simulink library "Control_Lib"  (R2018a)
settings: Solver=VariableStepAuto  StartTime=0.0  StopTime=10.0  RelTol=1e-3
undefined symbols (not defined in the file or in its folder): fb, Theta0, Tr_PLL
libraries: $bdroot x2, simulink x2
settings Model: Creator=Frederic_Colas  LastModifiedBy=fcolas

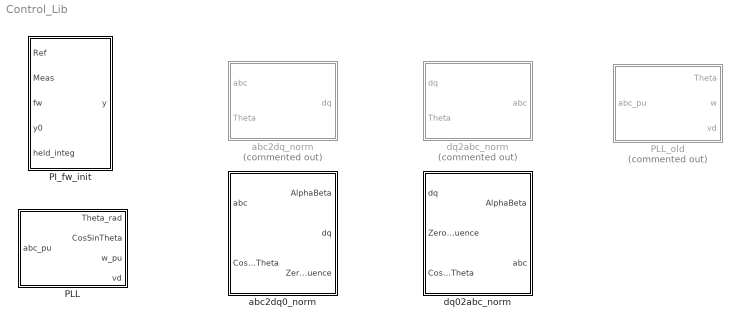
== system Control_Lib ==
  PI_fw_init : Subsystem  TreatAsAtomicUnit=on  mask{Kp=1, Ki=1}
  PLL : Subsystem  TreatAsAtomicUnit=on  mask{fb=fb, Tr_PLL=Tr_PLL, Theta0=Theta0}
      mask prompts: fb "fb (Hz)"; Tr_PLL "PLL time response (ms)"; Theta0 "Theta0 (°)"
      mask init:
      | wb = 2*pi*fb;
      | wn_PLL=5/(Tr_PLL/1000);
      | zeta_PLL = 1;
      | Kp_PLL = 2*zeta_PLL*wn_PLL/wb;
      | Ki_PLL = wn_PLL^2/wb;
  PLL_old : Subsystem  Commented=on  TreatAsAtomicUnit=on  mask{fb=50, Tr_PLL=10, zeta_PLL=1, Theta0=0}
      mask prompts: fb "fb (Hz)"; Tr_PLL "PLL time response (ms)"; zeta_PLL "Damping factor"; Theta0 "Theta0 (°)"
      mask init:
      | wb = 2*pi*fb;
      | wn_PLL=5/(Tr_PLL/1000);
      | zeta_PLL = 1;
      | Kp_PLL = 2*zeta_PLL*wn_PLL/wb;
      | Ki_PLL = wn_PLL^2/wb;
  abc2dq0_norm : Subsystem  TreatAsAtomicUnit=on  mask{referenceAxisMode=Reference axis at 90 degrees behind phase_a, baseUpdateGain=1/sqrt(3)}
      mask prompts: referenceAxisMode "Chosse reference axis of the angular position"; baseUpdateGain "Gain to update base from abc to dq0 frames"
      mask init:
      | Concordia33 = sqrt(2/3)*[[cos(0) cos(-2*pi/3) cos(-4*pi/3)];
      |                  [-sin(0) -sin(-2*pi/3) -sin(-4*pi/3)];
      |                  [1/sqrt(2) 1/sqrt(2) 1/sqrt(2)];];
      |              
      | Concordia33_inv = transpose(Concordia33);
      mask TypeOptions referenceAxisMode: Reference axis on phase_a | Reference axis at 90 degrees behind phase_a
      mask DialogControl DescGroupVar Prompt: CONFIGURATION
      mask DialogControl Container3 Prompt: Reference axis
      mask DialogControl Container4 Prompt: Base definition
      mask DialogControl Control1 Prompt: Gain = 1.0 : No base update
      mask DialogControl Control1_copy Prompt: Gain = 1/sqrt(3) : 1pu RMS in abc frame = 1pu in dq0 frame
  abc2dq_norm : Subsystem  Commented=on  TreatAsAtomicUnit=on
      mask DialogControl Control2 Prompt: abc to dq transformation with a normalization gain
  dq02abc_norm : Subsystem  TreatAsAtomicUnit=on  mask{referenceAxisMode=Reference axis at 90 degrees behind phase_a, baseUpdateGain=sqrt(3)}
      mask prompts: referenceAxisMode "Chosse reference axis of the angular position"; baseUpdateGain "Gain to update base from dq0 to abc frames"
      mask init: same as Control_Lib/abc2dq0_norm
      mask TypeOptions referenceAxisMode: Reference axis on phase_a | Reference axis at 90 degrees behind phase_a
      mask DialogControl DescGroupVar Prompt: CONFIGURATION
      mask DialogControl Container3 Prompt: Reference axis
      mask DialogControl Container4 Prompt: Base definition
      mask DialogControl Control1 Prompt: Gain = 1.0 : No base update
      mask DialogControl Control1_copy Prompt: Gain = sqrt(3) : 1pu in dq0 frame = 1pu RMS in abc frame
  dq2abc_norm : Subsystem  Commented=on  TreatAsAtomicUnit=on
      mask DialogControl Control2 Prompt: (Add text here)

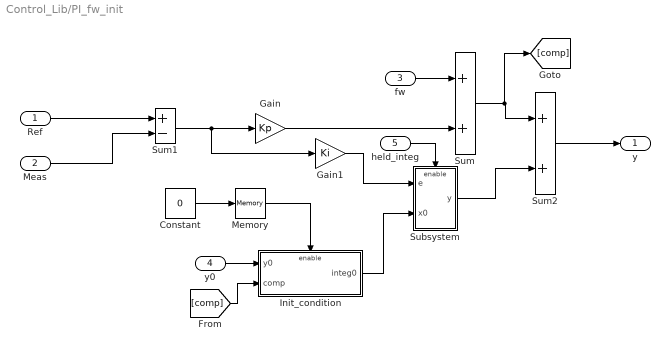
== system Control_Lib/PI_fw_init ==
  Ref : Inport
  Meas : Inport  Port=2
  fw : Inport  Port=3
  y0 : Inport  Port=4
  held_integ : Inport  Port=5
  Constant : Constant  Value=0
  Gain : Gain  Gain=Kp
  Gain1 : Gain  Gain=Ki
  Init_condition : Subsystem
  Memory : Memory  InitialCondition=1
  Subsystem : Subsystem
  Sum : Sum
  Sum1 : Sum  Inputs=+-
  Sum2 : Sum
  y : Outport  VectorParamsAs1DForOutWhenUnconnected=off
  wires:
  Gain/1 -> Sum/2
  fw/1 -> Sum/1
  Memory/1 -> Init_condition/Enable
  Constant/1 -> Memory/1
  y0/1 -> Init_condition/1(y0)
  Sum2/1 -> y/1
  Sum1/1 -> Gain1/1, Gain/1
  Sum/1 -> [comp], Sum2/1
  Meas/1 -> Sum1/2
  Ref/1 -> Sum1/1
  [comp] -> Init_condition/2(comp)
  Gain1/1 -> Subsystem/1(e)
  Init_condition/1(integ0) -> Subsystem/2(x0)
  Subsystem/1(y) -> Sum2/2
  held_integ/1 -> Subsystem/Enable

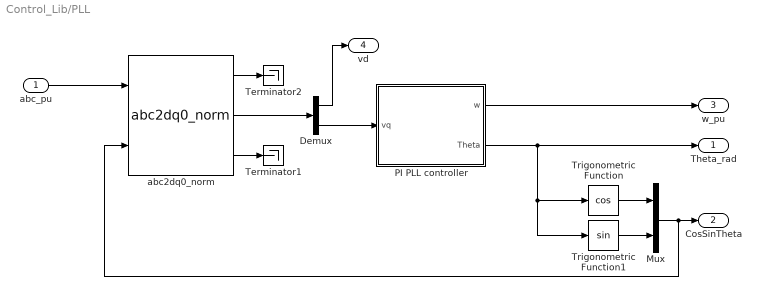
== system Control_Lib/PLL ==
  abc_pu : Inport
  Demux : Demux  Outputs=[1 1]
  Mux : Mux  Inputs=2
  PI PLL controller : Subsystem
  Terminator1 : Terminator
  Terminator2 : Terminator
  Trigonometric Function : Trigonometry  Operator=cos
  Trigonometric Function1 : Trigonometry
  abc2dq0_norm : $bdroot/abc2dq0_norm  referenceAxisMode=Reference axis at 90 degrees behind phase_a  baseUpdateGain=1/sqrt(3)
  Theta_rad : Outport  PortDimensions=1  VectorParamsAs1DForOutWhenUnconnected=off
  CosSinTheta : Outport  Port=2  PortDimensions=2  VectorParamsAs1DForOutWhenUnconnected=off
  w_pu : Outport  Port=3  PortDimensions=1  VectorParamsAs1DForOutWhenUnconnected=off
  vd : Outport  Port=4  PortDimensions=1  VectorParamsAs1DForOutWhenUnconnected=off
  wires:
  abc2dq0_norm/1 -> Terminator2/1
  abc2dq0_norm/3 -> Terminator1/1
  abc_pu/1 -> abc2dq0_norm/1
  Mux/1 -> CosSinTheta/1, abc2dq0_norm/2
  Trigonometric Function/1 -> Mux/1
  Trigonometric Function1/1 -> Mux/2
  PI PLL controller/2(Theta) -> Theta_rad/1, Trigonometric Function/1, Trigonometric Function1/1
  abc2dq0_norm/2 -> Demux/1
  PI PLL controller/1(w) -> w_pu/1
  Demux/2 -> PI PLL controller/1(vq)
  Demux/1 -> vd/1

== system Control_Lib/PLL_old ==
  abc_pu : Inport
  Demux : Demux  Outputs=2
  PI PLL controller : Subsystem
  abc2dq_norm : $bdroot/abc2dq_norm
  Theta : Outport  VectorParamsAs1DForOutWhenUnconnected=off
  w : Outport  Port=2  VectorParamsAs1DForOutWhenUnconnected=off
  vd : Outport  Port=3  VectorParamsAs1DForOutWhenUnconnected=off
  wires:
  abc2dq_norm/1 -> Demux/1
  abc_pu/1 -> abc2dq_norm/1
  PI PLL controller/2(Theta) -> abc2dq_norm/2, Theta/1
  Demux/1 -> vd/1
  PI PLL controller/1(w) -> w/1
  Demux/2 -> PI PLL controller/1(vq)

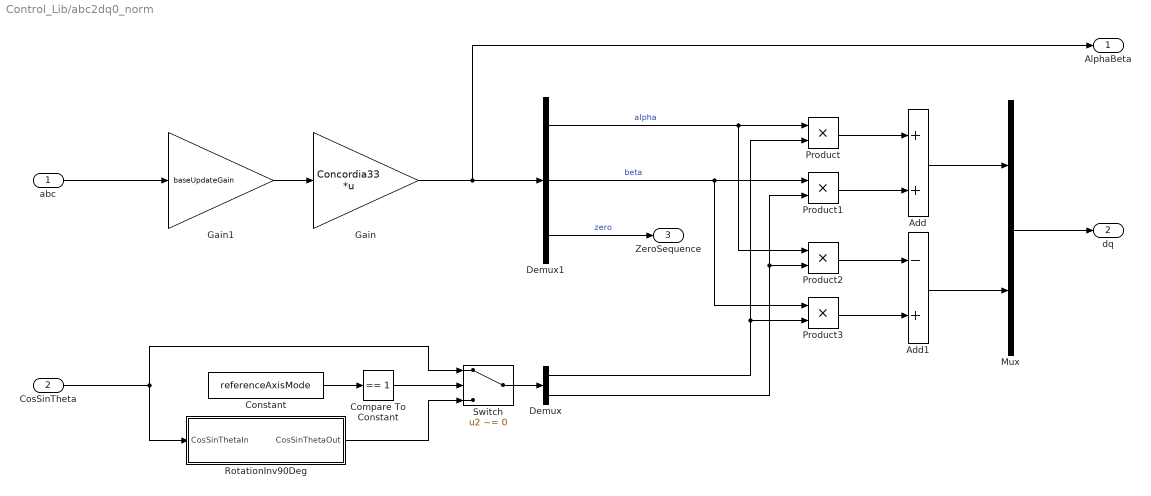
== system Control_Lib/abc2dq0_norm ==
  abc : Inport
  CosSinTheta : Inport  Port=2
  Add : Sum
  Add1 : Sum  Inputs=-+
  Compare To Constant : simulink/Logic and Bit Operations/Compare To Constant  relop===  const=1  OutDataTypeStr=boolean
  Constant : Constant  Value=referenceAxisMode  OutDataTypeStr=uint16
  Demux : Demux  Outputs=2
  Demux1 : Demux  Outputs=3
  Gain : Gain  Gain=Concordia33  Multiplication=Matrix(K*u)
  Gain1 : Gain  Gain=baseUpdateGain
  Mux : Mux  Inputs=2
  Product{,1..3} (4 alike) : Product
  RotationInv90Deg : Subsystem  VariantControl=ROTATIONINV90DEG
  Switch : Switch  Criteria=u2 ~= 0
  AlphaBeta : Outport  VectorParamsAs1DForOutWhenUnconnected=off
  dq : Outport  Port=2  VectorParamsAs1DForOutWhenUnconnected=off
  ZeroSequence : Outport  Port=3  VectorParamsAs1DForOutWhenUnconnected=off
  wires:
  abc/1 -> Gain1/1
  Product2/1 -> Add1/1
  Product/1 -> Add/1
  Demux1/1 -> Product/1, Product2/1  "alpha"
  Add/1 -> Mux/1
  Demux1/3 -> ZeroSequence/1  "zero"
  Mux/1 -> dq/1
  Demux1/2 -> Product1/1, Product3/1  "beta"
  Gain/1 -> AlphaBeta/1, Demux1/1
  Add1/1 -> Mux/2
  Demux/2 -> Product2/2, Product1/2
  Product1/1 -> Add/2
  Product3/1 -> Add1/2
  Demux/1 -> Product3/2, Product/2
  Switch/1 -> Demux/1
  CosSinTheta/1 -> Switch/1, RotationInv90Deg/1(CosSinThetaIn)
  RotationInv90Deg/1(CosSinThetaOut) -> Switch/3
  Constant/1 -> Compare To Constant/1
  Compare To Constant/1 -> Switch/2
  Gain1/1 -> Gain/1

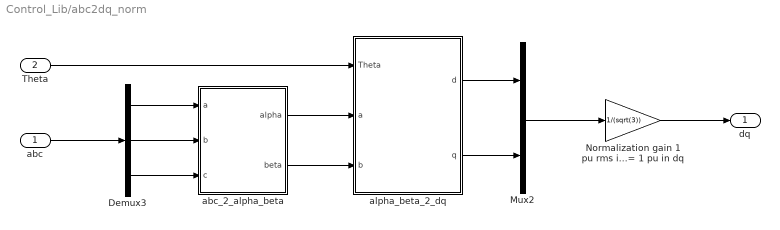
== system Control_Lib/abc2dq_norm ==
  abc : Inport
  Theta : Inport  Port=2
  Demux3 : Demux  Outputs=3
  Mux2 : Mux  Inputs=2
  Normalization gain 1 pu rms in abc = 1 pu in dq : Gain  Gain=1/(sqrt(3))
  abc_2_alpha_beta : Subsystem
  alpha_beta_2_dq : Subsystem
  dq : Outport  VectorParamsAs1DForOutWhenUnconnected=off
  wires:
  Normalization gain 1 pu rms in abc = 1 pu in dq/1 -> dq/1
  Theta/1 -> alpha_beta_2_dq/1(Theta)
  Demux3/3 -> abc_2_alpha_beta/3(c)
  abc/1 -> Demux3/1
  alpha_beta_2_dq/2(q) -> Mux2/2
  abc_2_alpha_beta/2(beta) -> alpha_beta_2_dq/3(b)
  alpha_beta_2_dq/1(d) -> Mux2/1
  Demux3/2 -> abc_2_alpha_beta/2(b)
  Demux3/1 -> abc_2_alpha_beta/1(a)
  abc_2_alpha_beta/1(alpha) -> alpha_beta_2_dq/2(a)
  Mux2/1 -> Normalization gain 1 pu rms in abc = 1 pu in dq/1

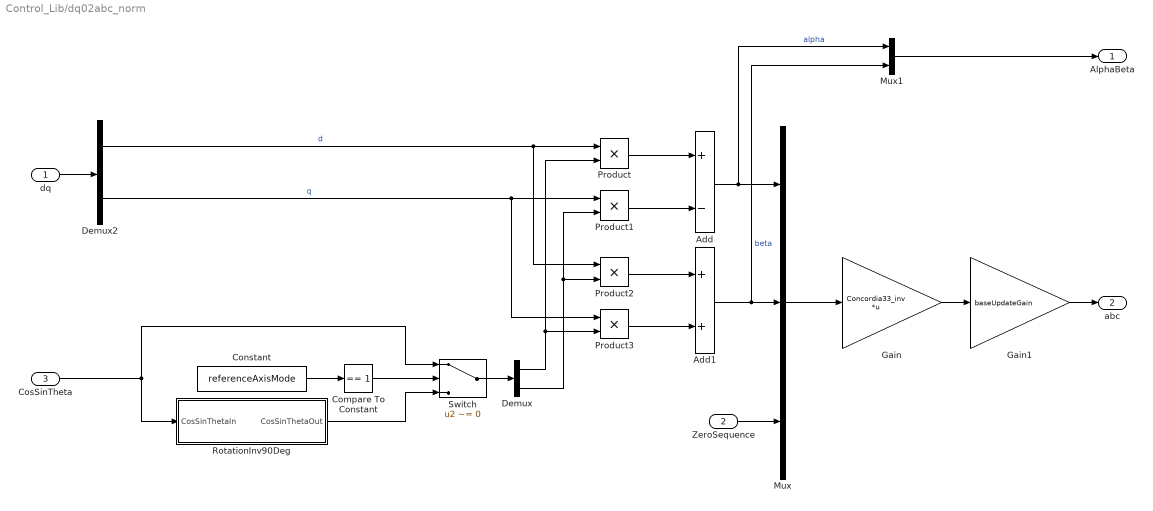
== system Control_Lib/dq02abc_norm ==
  dq : Inport
  ZeroSequence : Inport  Port=2
  CosSinTheta : Inport  Port=3
  Add : Sum  Inputs=+-
  Add1 : Sum
  Compare To Constant : simulink/Logic and Bit Operations/Compare To Constant  relop===  const=1  OutDataTypeStr=boolean
  Constant : Constant  Value=referenceAxisMode  OutDataTypeStr=uint16
  Demux : Demux  Outputs=2
  Demux2 : Demux  Outputs=2
  Gain : Gain  Gain=Concordia33_inv  Multiplication=Matrix(K*u)
  Gain1 : Gain  Gain=baseUpdateGain
  Mux : Mux  Inputs=3
  Mux1 : Mux  Inputs=2
  Product{,1..3} (4 alike) : Product
  RotationInv90Deg : Subsystem  VariantControl=ROTATIONINV90DEG
  Switch : Switch  Criteria=u2 ~= 0
  AlphaBeta : Outport  VectorParamsAs1DForOutWhenUnconnected=off
  abc : Outport  Port=2  VectorParamsAs1DForOutWhenUnconnected=off
  wires:
  Gain/1 -> Gain1/1
  Add/1 -> Mux1/1, Mux/1  "alpha"
  Demux2/1 -> Product2/1, Product/1  "d"
  ZeroSequence/1 -> Mux/3
  dq/1 -> Demux2/1
  CosSinTheta/1 -> RotationInv90Deg/1(CosSinThetaIn), Switch/1
  Product3/1 -> Add1/2
  Product2/1 -> Add1/1
  Compare To Constant/1 -> Switch/2
  Product1/1 -> Add/2
  Add1/1 -> Mux1/2, Mux/2  "beta"
  Demux2/2 -> Product3/1, Product1/1  "q"
  Product/1 -> Add/1
  Mux1/1 -> AlphaBeta/1
  Demux/2 -> Product1/2, Product2/2
  Switch/1 -> Demux/1
  Mux/1 -> Gain/1
  Demux/1 -> Product/2, Product3/2
  RotationInv90Deg/1(CosSinThetaOut) -> Switch/3
  Constant/1 -> Compare To Constant/1
  Gain1/1 -> abc/1

== system Control_Lib/dq2abc_norm ==
  dq : Inport
  Theta : Inport  Port=2
  Demux2 : Demux  Outputs=2
  Normalization gain 1 pu in dq = 1 pu rms in abc : Gain  Gain=sqrt(3)
  alpha_beta_2_abc : Subsystem
  dq_2_alpha_beta : Subsystem
  abc : Outport  VectorParamsAs1DForOutWhenUnconnected=off
  wires:
  dq_2_alpha_beta/1(a) -> alpha_beta_2_abc/1(a)
  dq_2_alpha_beta/2(b) -> alpha_beta_2_abc/2(b)
  Demux2/1 -> dq_2_alpha_beta/2(d)
  Demux2/2 -> dq_2_alpha_beta/3(q)
  Theta/1 -> dq_2_alpha_beta/1(Theta)
  dq/1 -> Normalization gain 1 pu in dq = 1 pu rms in abc/1
  alpha_beta_2_abc/1(abc) -> abc/1
  Normalization gain 1 pu in dq = 1 pu rms in abc/1 -> Demux2/1

== system Control_Lib/PI_fw_init/Init_condition ==
  y0 : Inport
  comp : Inport  Port=2
  Enable : EnablePort
  Sum : Sum  Inputs=-+
  integ0 : Outport  VectorParamsAs1DForOutWhenUnconnected=off
  wires:
  comp/1 -> Sum/1
  y0/1 -> Sum/2
  Sum/1 -> integ0/1

== system Control_Lib/PI_fw_init/Subsystem ==
  e : Inport
  x0 : Inport  Port=2
  Enable : EnablePort
  Integrator : Integrator  InitialConditionSource=external
  y : Outport  VectorParamsAs1DForOutWhenUnconnected=off
  wires:
  e/1 -> Integrator/1
  Integrator/1 -> y/1
  x0/1 -> Integrator/2

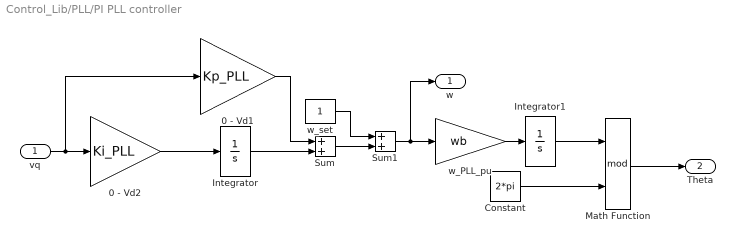
== system Control_Lib/PLL/PI PLL controller ==
  vq : Inport
  0 - Vd1 : Gain  Gain=Kp_PLL  SaturateOnIntegerOverflow=on  OutDataTypeStr=Inherit: Same as input  ParamDataTypeStr=Inherit: Same as input
  0 - Vd2 : Gain  Gain=Ki_PLL  SaturateOnIntegerOverflow=on  OutDataTypeStr=Inherit: Same as input  ParamDataTypeStr=Inherit: Same as input
  Constant : Constant  Value=2*pi
  Integrator : Integrator
  Integrator1 : Integrator  InitialCondition=Theta0*pi/180
  Math Function : Math  Operator=mod  SaturateOnIntegerOverflow=on
  Sum : Sum  SaturateOnIntegerOverflow=on
  Sum1 : Sum  SaturateOnIntegerOverflow=on
  w_PLL_pu : Gain  Gain=wb  SaturateOnIntegerOverflow=on  OutDataTypeStr=Inherit: Same as input  ParamDataTypeStr=Inherit: Same as input
  w_set : Constant
  w : Outport  VectorParamsAs1DForOutWhenUnconnected=off
  Theta : Outport  Port=2  VectorParamsAs1DForOutWhenUnconnected=off
  wires:
  Sum1/1 -> w_PLL_pu/1, w/1
  vq/1 -> 0 - Vd1/1, 0 - Vd2/1
  0 - Vd1/1 -> Sum/1
  Sum/1 -> Sum1/2
  Integrator/1 -> Sum/2
  w_PLL_pu/1 -> Integrator1/1
  w_set/1 -> Sum1/1
  0 - Vd2/1 -> Integrator/1
  Integrator1/1 -> Math Function/1
  Math Function/1 -> Theta/1
  Constant/1 -> Math Function/2

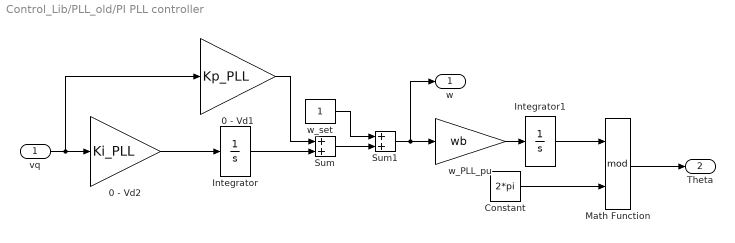
== system Control_Lib/PLL_old/PI PLL controller ==
  vq : Inport
  0 - Vd1 : Gain  Gain=Kp_PLL  SaturateOnIntegerOverflow=on  OutDataTypeStr=Inherit: Same as input  ParamDataTypeStr=Inherit: Same as input
  0 - Vd2 : Gain  Gain=Ki_PLL  SaturateOnIntegerOverflow=on  OutDataTypeStr=Inherit: Same as input  ParamDataTypeStr=Inherit: Same as input
  Constant : Constant  Value=2*pi
  Integrator : Integrator
  Integrator1 : Integrator  InitialCondition=Theta0*pi/180
  Math Function : Math  Operator=mod  SaturateOnIntegerOverflow=on
  Sum : Sum  SaturateOnIntegerOverflow=on
  Sum1 : Sum  SaturateOnIntegerOverflow=on
  w_PLL_pu : Gain  Gain=wb  SaturateOnIntegerOverflow=on  OutDataTypeStr=Inherit: Same as input  ParamDataTypeStr=Inherit: Same as input
  w_set : Constant
  w : Outport  VectorParamsAs1DForOutWhenUnconnected=off
  Theta : Outport  Port=2  VectorParamsAs1DForOutWhenUnconnected=off
  wires:
  Sum1/1 -> w_PLL_pu/1, w/1
  vq/1 -> 0 - Vd1/1, 0 - Vd2/1
  0 - Vd1/1 -> Sum/1
  Sum/1 -> Sum1/2
  Integrator/1 -> Sum/2
  w_PLL_pu/1 -> Integrator1/1
  w_set/1 -> Sum1/1
  0 - Vd2/1 -> Integrator/1
  Integrator1/1 -> Math Function/1
  Math Function/1 -> Theta/1
  Constant/1 -> Math Function/2

== system Control_Lib/abc2dq0_norm/RotationInv90Deg ==
  CosSinThetaIn : Inport
  Demux : Demux  Outputs=2
  Gain1 : Gain  Gain=-1
  Mux : Mux  Inputs=2
  CosSinThetaOut : Outport  VectorParamsAs1DForOutWhenUnconnected=off
  wires:
  Mux/1 -> CosSinThetaOut/1
  CosSinThetaIn/1 -> Demux/1
  Demux/1 -> Gain1/1
  Demux/2 -> Mux/1
  Gain1/1 -> Mux/2

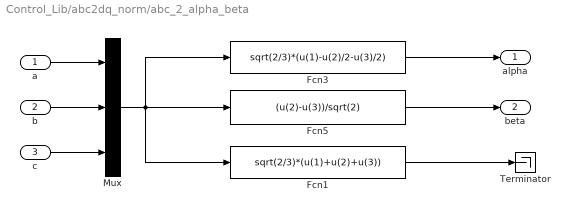
== system Control_Lib/abc2dq_norm/abc_2_alpha_beta ==
  a : Inport
  b : Inport  Port=2
  c : Inport  Port=3
  Fcn1 : Fcn  Expr=sqrt(2/3)*(u(1)+u(2)+u(3))
  Fcn3 : Fcn  Expr=sqrt(2/3)*(u(1)-u(2)/2-u(3)/2)
  Fcn5 : Fcn  Expr=(u(2)-u(3))/sqrt(2)
  Mux : Mux  Inputs=3
  Terminator : Terminator
  alpha : Outport  VectorParamsAs1DForOutWhenUnconnected=off
  beta : Outport  Port=2  VectorParamsAs1DForOutWhenUnconnected=off
  wires:
  Fcn5/1 -> beta/1
  Fcn3/1 -> alpha/1
  b/1 -> Mux/2
  a/1 -> Mux/1
  Mux/1 -> Fcn5/1, Fcn3/1, Fcn1/1
  Fcn1/1 -> Terminator/1
  c/1 -> Mux/3

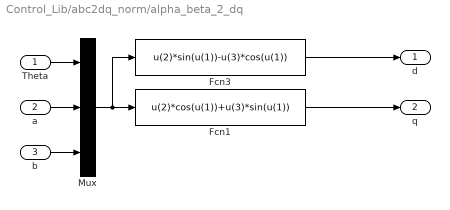
== system Control_Lib/abc2dq_norm/alpha_beta_2_dq ==
  Theta : Inport
  a : Inport  Port=2
  b : Inport  Port=3
  Fcn1 : Fcn  Expr=u(2)*cos(u(1))+u(3)*sin(u(1))
  Fcn3 : Fcn  Expr=u(2)*sin(u(1))-u(3)*cos(u(1))
  Mux : Mux  Inputs=3
  d : Outport  VectorParamsAs1DForOutWhenUnconnected=off
  q : Outport  Port=2  VectorParamsAs1DForOutWhenUnconnected=off
  wires:
  Fcn1/1 -> q/1
  Fcn3/1 -> d/1
  b/1 -> Mux/3
  a/1 -> Mux/2
  Mux/1 -> Fcn1/1, Fcn3/1
  Theta/1 -> Mux/1

== system Control_Lib/dq02abc_norm/RotationInv90Deg ==
  CosSinThetaIn : Inport
  Demux1 : Demux  Outputs=2
  Gain1 : Gain  Gain=-1
  Mux1 : Mux  Inputs=2
  CosSinThetaOut : Outport  VectorParamsAs1DForOutWhenUnconnected=off
  wires:
  Gain1/1 -> Mux1/2
  Demux1/1 -> Gain1/1
  Mux1/1 -> CosSinThetaOut/1
  CosSinThetaIn/1 -> Demux1/1
  Demux1/2 -> Mux1/1

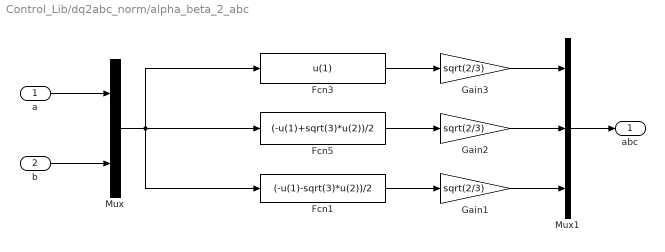
== system Control_Lib/dq2abc_norm/alpha_beta_2_abc ==
  a : Inport
  b : Inport  Port=2
  Fcn1 : Fcn  Expr=(-u(1)-sqrt(3)*u(2))/2
  Fcn3 : Fcn  Expr=u(1)
  Fcn5 : Fcn  Expr=(-u(1)+sqrt(3)*u(2))/2
  Gain1 : Gain  Gain=sqrt(2/3)
  Gain2 : Gain  Gain=sqrt(2/3)
  Gain3 : Gain  Gain=sqrt(2/3)
  Mux : Mux  Inputs=2
  Mux1 : Mux  Inputs=[1 1 1]
  abc : Outport  VectorParamsAs1DForOutWhenUnconnected=off
  wires:
  Mux/1 -> Fcn3/1, Fcn5/1, Fcn1/1
  a/1 -> Mux/1
  b/1 -> Mux/2
  Fcn3/1 -> Gain3/1
  Fcn5/1 -> Gain2/1
  Fcn1/1 -> Gain1/1
  Gain1/1 -> Mux1/3
  Gain2/1 -> Mux1/2
  Gain3/1 -> Mux1/1
  Mux1/1 -> abc/1

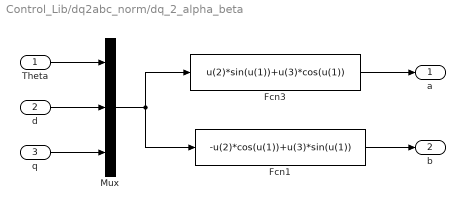
== system Control_Lib/dq2abc_norm/dq_2_alpha_beta ==
  Theta : Inport
  d : Inport  Port=2
  q : Inport  Port=3
  Fcn1 : Fcn  Expr=-u(2)*cos(u(1))+u(3)*sin(u(1))
  Fcn3 : Fcn  Expr=u(2)*sin(u(1))+u(3)*cos(u(1))
  Mux : Mux  Inputs=3
  a : Outport  VectorParamsAs1DForOutWhenUnconnected=off
  b : Outport  Port=2  VectorParamsAs1DForOutWhenUnconnected=off
  wires:
  Fcn1/1 -> b/1
  Fcn3/1 -> a/1
  q/1 -> Mux/3
  d/1 -> Mux/2
  Theta/1 -> Mux/1
  Mux/1 -> Fcn3/1, Fcn1/1
